simulink model "motorcontroller"  (R2020b)
settings: Solver=FixedStepAuto  StartTime=0.0  StopTime=Endtime  FixedStep=0.05  RelTol=1e-3
values from neighbouring files (symbols this model uses):
  Kd = 0    [ControllerModel_2020.m]
  Ki = 0.1    [ControllerModel_2020.m]
  Kp = 0.1    [ControllerModel_2020.m]
  SV = 1000    [ControllerModel_2020.m]
libraries: MBDLib_2020 x4
settings Model: Creator=005274  LastModifiedBy=005274

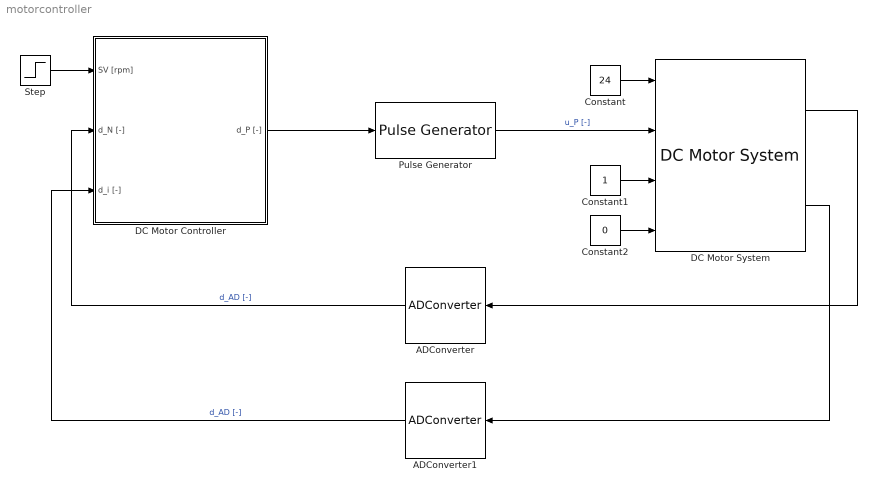
== system motorcontroller ==
  ADConverter : MBDLib_2020/Interface/ADConverter  n=10  V_max=5  V_min=0
      settings: SourceProductName=MBDLibrary
  ADConverter1 : MBDLib_2020/Interface/ADConverter  n=10  V_max=5  V_min=0
      settings: SourceProductName=MBDLibrary
  Constant : Constant  Value=24
  Constant1 : Constant
  Constant2 : Constant  Value=0
  DC Motor Controller : Subsystem
  "DC Motor System " : MBDLib_2020/Plant/DC Motor System  SystemSampleTime=-1  VariantActivationTime=update diagram  Latency=0  AutoFrameSizeCalculation=off
      settings: SourceProductName=MBDLibrary
  "Pulse Generator " : MBDLib_2020/Interface/Pulse Generator  n=8
      settings: SourceProductName=MBDLibrary
  Step : Step  After=SV  SampleTime=0
  wires:
  DC Motor Controller/1(d_P [-]) -> "Pulse Generator "/1
  "Pulse Generator "/1 -> "DC Motor System "/2  "u_P [-]"
  Constant/1 -> "DC Motor System "/1
  Constant1/1 -> "DC Motor System "/3
  Constant2/1 -> "DC Motor System "/4
  "DC Motor System "/2 -> ADConverter1/1
  "DC Motor System "/1 -> ADConverter/1
  ADConverter1/1 -> DC Motor Controller/3(d_i [-])  "d_AD [-]"
  ADConverter/1 -> DC Motor Controller/2(d_N [-])  "d_AD [-]"
  Step/1 -> DC Motor Controller/1(SV [rpm])

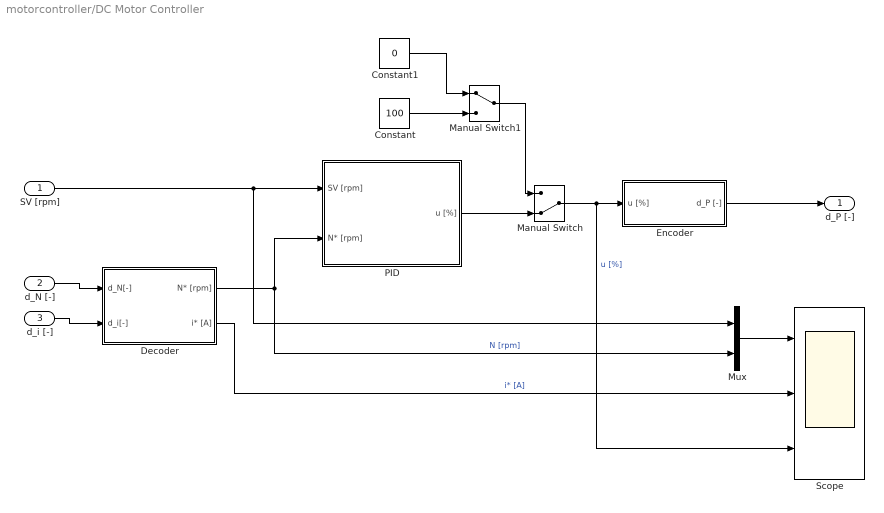
== system motorcontroller/DC Motor Controller ==
  SV [rpm] : Inport
  d_N [-] : Inport  Port=2
  d_i [-] : Inport  Port=3
  Constant : Constant  Value=100
  Constant1 : Constant  Value=0
  Decoder : Subsystem
  Encoder : Subsystem
  Manual Switch : ManualSwitch  CurrentSetting=0
  Manual Switch1 : ManualSwitch
  Mux : Mux  Inputs=2
  PID : Subsystem
  Scope : Scope  NumInputPorts=3
  d_P [-] : Outport
  wires:
  PID/1(u [%]) -> Manual Switch/2
  Decoder/2(i* [A]) -> Scope/2  "i* [A]"
  Decoder/1(N* [rpm]) -> PID/2(N* [rpm]), Mux/2  "N [rpm]"
  Constant1/1 -> Manual Switch1/1
  Manual Switch1/1 -> Manual Switch/1
  SV [rpm]/1 -> Mux/1, PID/1(SV [rpm])
  Manual Switch/1 -> Scope/3, Encoder/1(u [%])  "u [%]"
  Encoder/1(d_P [-]) -> d_P [-]/1
  d_i [-]/1 -> Decoder/2(d_i[-])
  d_N [-]/1 -> Decoder/1(d_N[-])
  Mux/1 -> Scope/1
  Constant/1 -> Manual Switch1/2

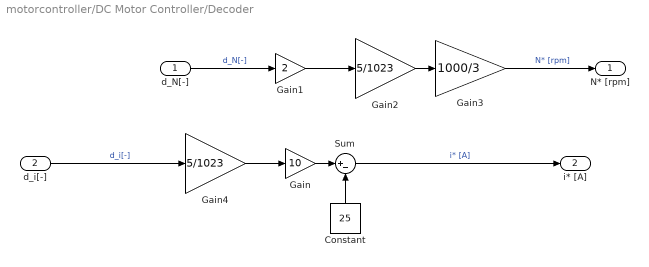
== system motorcontroller/DC Motor Controller/Decoder ==
  d_N[-] : Inport
  d_i[-] : Inport  Port=2
  Constant : Constant  Value=25
  Gain : Gain  Gain=10
  Gain1 : Gain  Gain=2
  Gain2 : Gain  Gain=5/1023
  Gain3 : Gain  Gain=1000/3
  Gain4 : Gain  Gain=5/1023
  Sum : Sum  Inputs=|+-
  N* [rpm] : Outport
  i* [A] : Outport  Port=2
  wires:
  Gain/1 -> Sum/1
  Constant/1 -> Sum/2
  d_i[-]/1 -> Gain4/1  "d_i[-]"
  Sum/1 -> i* [A]/1  "i* [A]"
  Gain1/1 -> Gain2/1
  d_N[-]/1 -> Gain1/1  "d_N[-]"
  Gain2/1 -> Gain3/1
  Gain3/1 -> N* [rpm]/1  "N* [rpm]"
  Gain4/1 -> Gain/1

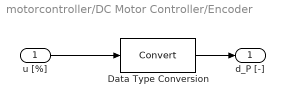
== system motorcontroller/DC Motor Controller/Encoder ==
  u [%] : Inport
  Data Type Conversion : DataTypeConversion
  d_P [-] : Outport
  wires:
  Data Type Conversion/1 -> d_P [-]/1
  u [%]/1 -> Data Type Conversion/1

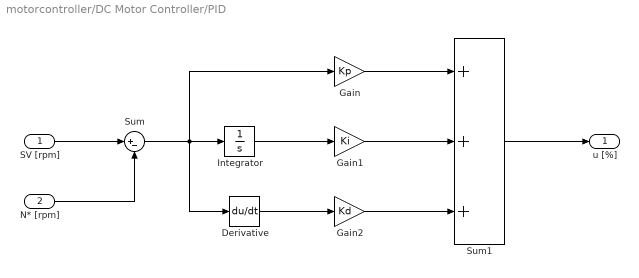
== system motorcontroller/DC Motor Controller/PID ==
  SV [rpm] : Inport
  N* [rpm] : Inport  Port=2
  Derivative : Derivative
  Gain : Gain  Gain=Kp
  Gain1 : Gain  Gain=Ki
  Gain2 : Gain  Gain=Kd
  Integrator : Integrator
  Sum : Sum  Inputs=|+-
  Sum1 : Sum  Inputs=+++
  u [%] : Outport
  wires:
  N* [rpm]/1 -> Sum/2
  SV [rpm]/1 -> Sum/1
  Sum/1 -> Derivative/1, Gain/1, Integrator/1
  Derivative/1 -> Gain2/1
  Integrator/1 -> Gain1/1
  Gain1/1 -> Sum1/2
  Gain/1 -> Sum1/1
  Gain2/1 -> Sum1/3
  Sum1/1 -> u [%]/1
